simulink model "ISC_laboratorio_02_03"  (R2019a)
settings: Solver=FixedStepAuto  StartTime=0.0  StopTime=50  FixedStep=0.001  RelTol=1e-3
undefined symbols (not defined in the file): x0
settings Model: Creator=guilh  LastModifiedBy=guilh
settings DataIOCC: SaveOutput=off  ReturnWorkspaceOutputs=off  TimeSaveName=t

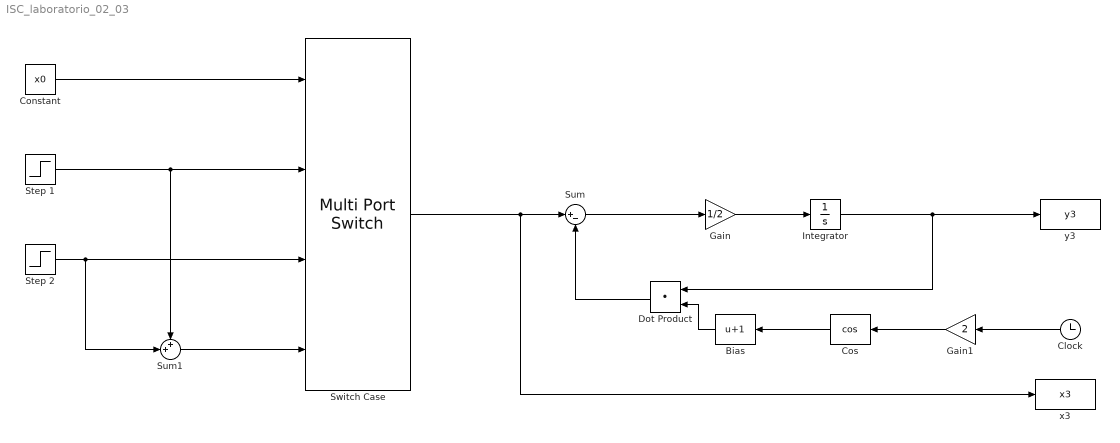
== system ISC_laboratorio_02_03 ==
  Bias : Bias  Bias=1
  Clock : Clock
  Constant : Constant  Value=x0
  Cos : Trigonometry  Operator=cos
  Dot Product : DotProduct  InputSameDT=on  OutDataTypeStr=Inherit: Inherit via internal rule
  Gain : Gain  Gain=1/2
  Gain1 : Gain  Gain=2
  Integrator : Integrator
  Step 1 : Step  Time=0  SampleTime=0
  Step 2 : Step  Time=0  After=2  SampleTime=0
  Sum : Sum  Inputs=|+-
  Sum1 : Sum  Inputs=++|
  Switch Case : MultiPortSwitch
  x3 : ToWorkspace  VariableName=x3  SampleTime=-1
  y3 : ToWorkspace  VariableName=y3  SampleTime=-1
  wires:
  Step 1/1 -> Sum1/1, Switch Case/2
  Constant/1 -> Switch Case/1
  Step 2/1 -> Sum1/2, Switch Case/3
  Sum1/1 -> Switch Case/4
  Clock/1 -> Gain1/1
  Gain1/1 -> Cos/1
  Cos/1 -> Bias/1
  Bias/1 -> Dot Product/2
  Integrator/1 -> Dot Product/1, y3/1
  Gain/1 -> Integrator/1
  Dot Product/1 -> Sum/2
  Switch Case/1 -> x3/1, Sum/1
  Sum/1 -> Gain/1
